simulink model "observer"  (R2022b)
settings: Solver=VariableStepAuto  StartTime=0.0  StopTime=200  RelTol=1e-3
undefined symbols (not defined in the file): A, B, C, L
settings Model: Creator=amoralesma  LastModifiedBy=amoralesma

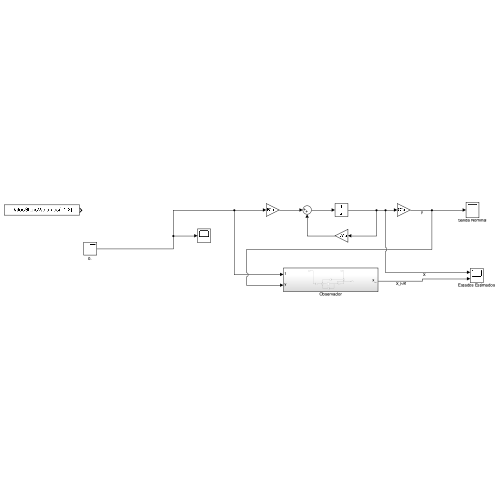
[thumbnail: Simulink's stored preview of the top-level diagram]
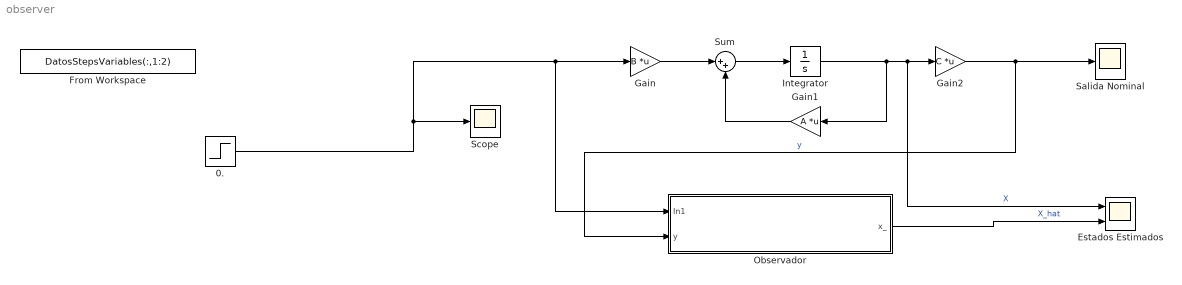
== system observer ==
  0. : Step  After=0.3  SampleTime=0
  Estados Estimados : Scope  NumInputPorts=2
  From Workspace : FromWorkspace  VariableName=DatosStepsVariables(:,1:2)  SampleTime=2.5e-3
  Gain : Gain  Gain=B  Multiplication=Matrix(K*u)
  Gain1 : Gain  Gain=A  Multiplication=Matrix(K*u)
  Gain2 : Gain  Gain=C  Multiplication=Matrix(K*u)
  Integrator : Integrator
  Observador : Subsystem
  Salida Nominal : Scope
  Scope : Scope
  Sum : Sum  Inputs=|++
  wires:
  Integrator/1 -> Gain1/1, Estados Estimados/1, Gain2/1  "X"
  Gain1/1 -> Sum/2
  Sum/1 -> Integrator/1
  Gain/1 -> Sum/1
  Gain2/1 -> Observador/2(y), Salida Nominal/1  "y"
  0./1 -> Observador/1(In1), Gain/1, Scope/1
  Observador/1(x_) -> Estados Estimados/2  "X_hat"

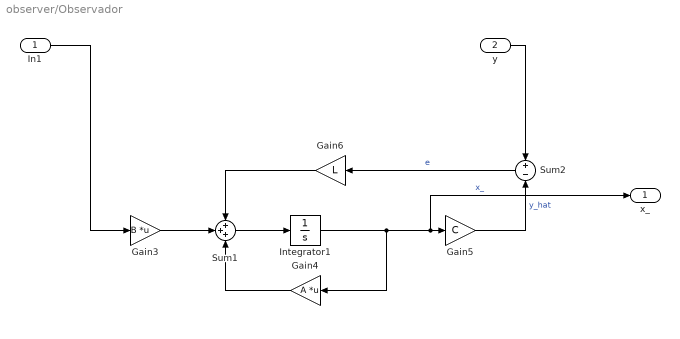
== system observer/Observador ==
  In1 : Inport
  y : Inport  Port=2
  Gain3 : Gain  Gain=B  Multiplication=Matrix(K*u)
  Gain4 : Gain  Gain=A  Multiplication=Matrix(K*u)
  Gain5 : Gain  Gain=C
  Gain6 : Gain  Gain=L
  Integrator1 : Integrator
  Sum1 : Sum  Inputs=+++
  Sum2 : Sum  Inputs=+|-
  x_ : Outport
  wires:
  In1/1 -> Gain3/1
  y/1 -> Sum2/1
  Gain5/1 -> Sum2/2  "y_hat"
  Sum1/1 -> Integrator1/1
  Gain3/1 -> Sum1/2
  Gain6/1 -> Sum1/1
  Integrator1/1 -> Gain4/1, x_/1, Gain5/1  "x_"
  Sum2/1 -> Gain6/1  "e"
  Gain4/1 -> Sum1/3
